simulink model "Requriment_44"  (R2021a)
settings: Solver=FixedStepDiscrete  StartTime=0.0  StopTime=50  FixedStep=1  RelTol=1e-3
undefined symbols (not defined in the file): amber, charged, critical_fault, red
libraries: simulink x8
settings Model: DataDictionary=soc.sldd  Creator=Rahul  LastModifiedBy=Rahul

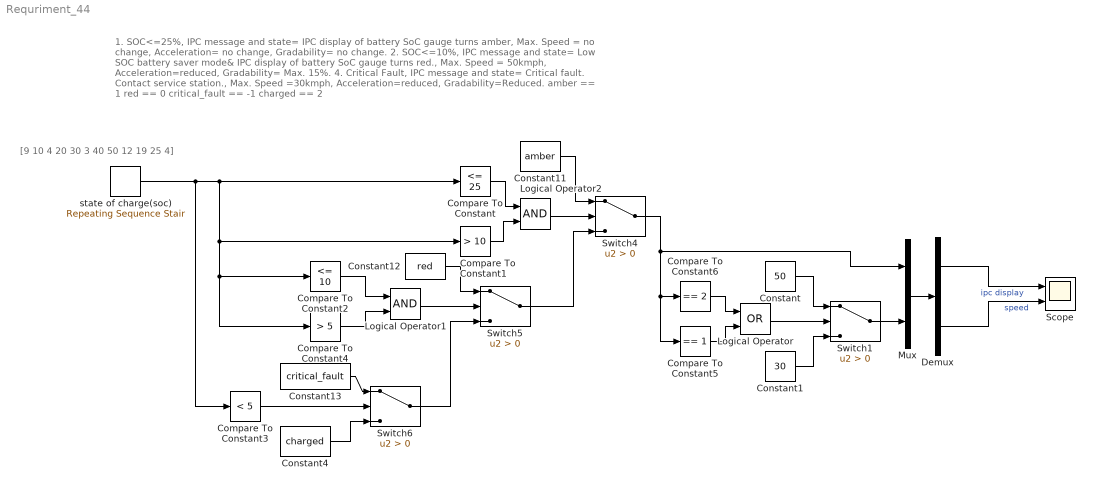
== system Requriment_44 ==
  note: [9 10 4 20 30 3 40 50 12 19 25 4]
  note: 1. SOC<=25%, IPC message and state= IPC display of battery SoC gauge turns amber, Max. Speed = no change, Acceleration= no change, Gradability= no change.
      | 2. SOC<=10%, IPC message and state= Low SOC battery saver mode& IPC display of battery SoC gauge turns red., Max. Speed = 50kmph, Acceleration=reduced, Gradability= Max. 15%.
      | 4. Critical Fault, IPC message and state= Critical fault. Contact service station., Max. Speed =30kmph, Acceleration=reduced, Gradability=Reduced.
      | amber == 1 red == 0 critical_fault == -1 charged == 2
  Compare To Constant : simulink/Logic and Bit Operations/Compare To Constant  relop=<=  const=25  OutDataTypeStr=boolean
  Compare To Constant1 : simulink/Logic and Bit Operations/Compare To Constant  relop=>  const=10  OutDataTypeStr=boolean
  Compare To Constant2 : simulink/Logic and Bit Operations/Compare To Constant  relop=<=  const=10  OutDataTypeStr=boolean
  Compare To Constant3 : simulink/Logic and Bit Operations/Compare To Constant  relop=<  const=5  OutDataTypeStr=boolean
  Compare To Constant4 : simulink/Logic and Bit Operations/Compare To Constant  relop=>  const=5  OutDataTypeStr=boolean
  Compare To Constant5 : simulink/Logic and Bit Operations/Compare To Constant  relop===  const=1  OutDataTypeStr=boolean
  Compare To Constant6 : simulink/Logic and Bit Operations/Compare To Constant  relop===  const=2  OutDataTypeStr=boolean
  Constant : Constant  Value=50
  Constant1 : Constant  Value=30
  Constant11 : Constant  Value=amber
  Constant12 : Constant  Value=red
  Constant13 : Constant  Value=critical_fault
  Constant4 : Constant  Value=charged
  Demux : Demux  Outputs=2
  Logical Operator : Logic  Operator=OR  AllPortsSameDT=off  OutDataTypeStr=boolean
  Logical Operator1 : Logic  AllPortsSameDT=off  OutDataTypeStr=boolean
  Logical Operator2 : Logic  AllPortsSameDT=off  OutDataTypeStr=boolean
  Mux : Mux  Inputs=2
  Scope : Scope  NumInputPorts=2
  Switch{1,4..6} (4 alike) : Switch  Criteria=u2 > Threshold
  state of charge(soc) : simulink/Sources/Repeating Sequence Stair  OutValues="[9 10 4 20 30 3 40  12 19 25 50 4]"  tsamp=-1  OutMin=[]  OutMax=[]  OutDataTypeStr=double  OutputDataTypeScalingMode=double  OutDataType=fixdt(0,8)  ConRadixGroup=Best Precision: Vector-wise  OutScaling=2^-12
  wires:
  state of charge(soc)/1 -> Compare To Constant3/1, Compare To Constant1/1, Compare To Constant4/1, Compare To Constant2/1, Compare To Constant/1
  Compare To Constant/1 -> Logical Operator2/1
  Compare To Constant1/1 -> Logical Operator2/2
  Logical Operator2/1 -> Switch4/2
  Constant11/1 -> Switch4/1
  Constant12/1 -> Switch5/1
  Compare To Constant3/1 -> Switch6/2
  Constant13/1 -> Switch6/1
  Constant4/1 -> Switch6/3
  Switch6/1 -> Switch5/3
  Switch5/1 -> Switch4/3
  Switch4/1 -> Mux/1, Compare To Constant6/1, Compare To Constant5/1
  Compare To Constant2/1 -> Logical Operator1/1
  Compare To Constant4/1 -> Logical Operator1/2
  Logical Operator1/1 -> Switch5/2
  Compare To Constant5/1 -> Logical Operator/2
  Logical Operator/1 -> Switch1/2
  Constant/1 -> Switch1/1
  Constant1/1 -> Switch1/3
  Switch1/1 -> Mux/2
  Compare To Constant6/1 -> Logical Operator/1
  Mux/1 -> Demux/1
  Demux/1 -> Scope/1  "ipc display"
  Demux/2 -> Scope/2  "speed"
